simulink model "A4_10_bodeExp"  (Simulink 7.4)
settings: Solver=FixedStepDiscrete  StartTime=0.0  StopTime=50  RelTol=1e-3
undefined symbols (not defined in the file or in its folder): frequency
libraries: DCmotor_library x1
settings Model: Creator=Natalia  LastModifiedBy=ma
settings DebuggingCC: StrictBusMsg=ErrorLevel1
settings CodeAppCC: CustomSymbolStrType=$N$R$M_T

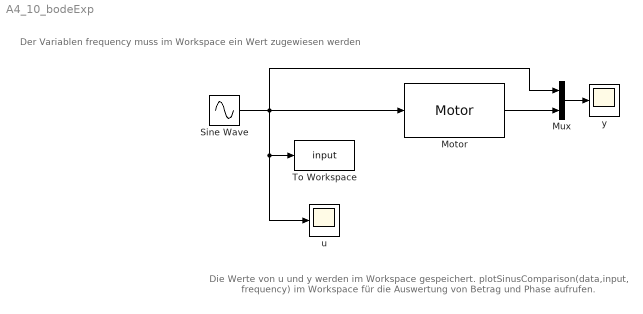
== system A4_10_bodeExp ==
  note: Die Werte von u und y werden im Workspace gespeichert.
      | plotSinusComparison(data,input, frequency) im Workspace
      | für die Auswertung von Betrag und Phase aufrufen.
  note: Der Variablen
      | frequency
      | muss im Workspace ein
      | Wert zugewiesen werden
  Motor : DCmotor_library/Motor  motoridinput=8  name_signal=Velocity  ts=10
  Mux : Mux  Inputs=2
  Sine Wave : Sin  Amplitude=2  Bias=3  Frequency=frequency  SampleTime=0
  To Workspace : ToWorkspace  VariableName=input  SampleTime=-1  SaveFormat=Structure With Time
  u : Scope
      settings: YMin=-0.5  YMax=11  SaveName=ScopeData2
  y : Scope
      settings: YMax=110
  wires:
  Sine Wave/1 -> Mux/1, u/1, To Workspace/1, Motor/1
  Mux/1 -> y/1
  Motor/1 -> Mux/2
